simulink model "CM660A_HwTq1Meas"  (R2013b)
settings: Solver=FixedStepDiscrete  StartTime=0.0  StopTime=20  FixedStep=0.002  RelTol=1e-3
undefined symbols (not defined in the file): ELECGLBPRM_HWTQOFFS_HWNWTMTR_F32, ELECGLBPRM_HWTQSATNLOWRLIM_HWNWTMTR_F32, ELECGLBPRM_HWTQSATNUPPRLIM_HWNWTMTR_F32, ELECGLBPRM_HWTQSCA_ULS_F32, ELECGLBPRM_NOFLT_CNT_U08, ELECGLBPRM_OFFSTRIMNOTPRFM_CNT_U08, ELECGLBPRM_PRTCLFLT_CNT_U08, ELECGLBPRM_SNSRINTFLT_CNT_U08, HwTq1MeasHwTq1PrtclFltFailStep, HwTq1MeasHwTq1PrtclFltPassStep, NtcNr1, NtcSts1, RACKLIMRCCWEOTSCA_ULS_F32, RACKLIMRCWEOTSCA_ULS_F32, sigbuilder_block, SigQlfr1
libraries: simulink x25, NxtrNvM x3, NxtrLim x2
(part 1 of 3)
settings Model: RequirementInfo={'doors' '00006115' '1' 'false' 'DOORS Surrogate Item' '' } %GIDa_184d7b6b_0c7e_41d3_b9a0_1a88eb3981d4  reqMgrSettings="100 S'doors','misc'{{S'surrogatepath','savemodel','savesurrogate','updateLinks','doorsLinks2sl','slLinks2Doors','purgeDoors','purgeSimulink','detaillevel','surrogateId','synctime'{{T\"/ESG Group/CM660A_HwTq1Meas\",M[1],M[1],M[0],M[0],M[1],M[0],M[0],M[1],T\"00006115\",T\"\"}},S'mode','pathStorage'{{T\"generic\",T\"modelRelative\"}}}}"  BufferReuse=off  Creator=CZ68DS  LastModifiedBy=TZBSJD
settings SolverCC: AutoInsertRateTranBlk=on
settings DataIOCC: SaveFormat=StructureWithTime
settings OptimizationCC: BlockReduction=off  DefaultUnderspecifiedDataType=single  OptimizeBlockIOStorage=off  BufferReuse=off  ExpressionFolding=off  LocalBlockOutputs=off  OptimizeModelRefInitCode=on  LifeSpan=1
settings DebuggingCC: MultiTaskDSMMsg=warning
settings HardwareCC: ProdIntDivRoundTo=Zero  ProdEndianess=LittleEndian  ProdHWDeviceType=Generic->Custom  TargetIntDivRoundTo=Zero  TargetEndianess=LittleEndian  TargetHWDeviceType=Generic->Custom
settings RTWCC: SystemTargetFile=ert.tlc  TemplateMakefile=ert_default_tmf  Description=Embedded Coder  ProcessScript=ert_make_rtw_hook
settings CodeAppCC: IgnoreCustomStorageClasses=off
settings ERTTargetCC: CodeReplacementLibrary=ANSI_C  GenerateSampleERTMain=on  ERTCustomFileTemplate=example_file_process.tlc

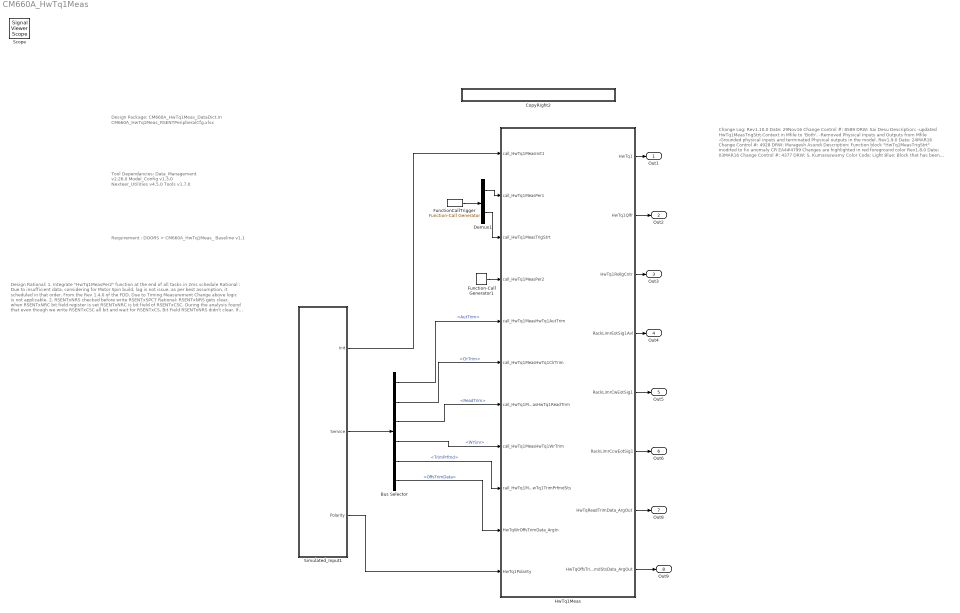
== system CM660A_HwTq1Meas ==
  note: Design Package:
      |
      | CM660A_HwTq1Meas_DataDict.m
      | CM660A_HwTq1Meas_RSENTPeripheralCfg.xlsx
  note: Change Log:
      | Rev1.10.0
      | Date: 29Nov16
      | Change Control #: 8589
      | DRW: Sai Desu
      | Description:
      | -updated HwTq1MeasTrigStrt.Context in Mfile to 'Both'.
      | -Removed Physical Inputs and Outputs from Mfile
      | -Grounded physical inputs and terminated Physical outputs in the model.
      |
      | Rev1.9.0
      | Date: 24MAR16
      | Change Control #: 4928
      | DRW: Muragesh Asundi
      | Description:
      | Function block "HwTq1MeasTrigStrt" modifed to fix anomaly CR EA4#4799
      | Changes are highlighted in red foreground color
      |
      | Rev1.8.0
      | Date: 03MAR16
      | Change Control #: 4377
      | DRW: S. Kumaraswamy
      | Color Code:
      | Light Blue:	Block that has been changed
      | 				Follow the color until the change is observed to the deepeset level
      | Dark Gray:	Client Call Blocks. Contents cannot be modified
      |
      | Rev1.7.0
      | Date: 19JAN2016
      | Change Control #: 3374
      | DRW: K. Patel
      | Description:
      | - Refer Red Color High lighted Changes.
      | - "CM660A_HwTq1Meas_RSENTPeripheralCfg.xlsx" change
      |
      | Rev1.6.0
      | Date: 16DEC2015
      | Change Control #: 3157
      | DRW: K. Patel
      | Description:
      | - Refer Red Color High lighted Changes.
      |
      | Rev: 1.5.0
      | Date: 23OCT2015
      | Change Control #: EA4#2217
      | DRW: K. Patel
      | Description:
      | - Slow Serial Message Fix
      | - EA4 Naming Correction for HwTq1MeasTrigStart
      |
      | Rev: 1.4.0
      | Date: 09OCT2015
      | Change Control #: EA4#1921
      | DRW: K. Patel
      | Description:
      | - Torque Trigger server function, Per3 change to Per2, Missing Message Counter add per1,
      | remove register from "CM660A_HwTq1Meas_RSENTPeripheralCfg.xlsx",
      | change sync time to 16
      |
      | Rev: 1.3.0
      | Date: 02OCT2015
      | Change Control #: EA4#1812
      | DRW: Pallav G/Muragesh A (KPIT)
      | Description:
      | - Corrected output signal names RickLimrCcwEotSig1,
      | RickLimrCwEotSig1 to RackLimrCcwEotSig1 and RackLimrCwEotSig1 respectively
      | - Range limiter added for above two output signals
      |
      | Rev: 1.2.0
      | Date: 20AUG2015
      | Change Control #: WCR-EA4#1285
      | DRW: K. Patel
      | Description:
      | - Rack Limiter End of Travel Signal 0 Data Read Function added
      |
      | Rev: 1.1.0
      | Date: 31JUL2015
      | Change Control #: WCR-EA4#1164
      | DRW: K. Patel
      | Description:
      | - m file correction, Tick Time change from 1us to 1.2us
      | - Global Constant
      |
      |
      | Rev: 1.0.0
      | Date: 30JUN2015
      | Change Control #: WCR-EA4#1028
      | DRW: K. Patel
      | Description:
      | - Initial Release
      | - Trim Services Added
      |
      | DRW: Keyur Patel
      | Description:
      | - Model intent to implement EA4 SENT1 based Digital Torque implementation for T1xx.
      |    model runs at three different function rate:
      |       1) Init - Configure Peripheral
      |       2) 2ms - Running SENT data, protocol fault, HwNm calculation, SENT trigger.
      |       3) 100ms - Per3 Trim Not Performed evaluation
      |       4) Event Trim Service - Auto, Clear, Write, Read, Trim Performed Status
      | - Fault Injection added
      | - Copyright Blocks added to each layer
  note: Tool Dependancies:
      |
      | Data_Management v2.26.0
      | Model_Config v1.3.0
      | Nexteer_Utilities v4.5.0
      | Tools v1.7.0
  note: Requirement :
      |
      | DOORS > CM660A_HwTq1Meas_ Baseline v1.1
  note: Design Rational:
      |
      | 1. Integrate "HwTq1MeasPer2" function at the end of all tasks in 2ms schedule
      | Rational : Due to insufficient data, considering for Motor Spin build, lag is not
      | issue, as per best assumption, it scheduled in that order.
      |
      | From the Rev 1.4.0 of the FDD, Due to Timing Measurement Change above logic
      | is not applicable.
      |
      | 2. RSENTxNRS checked before write RSENTxSPCT
      | Rational: RSENTxNRS gets clear, when RSENTxNRC bit field register is set
      | RSENTxNRC is bit field of RSENTxCSC. During the analysis found that
      | even though we write RSENTxCSC all bit and wait for RSENTxCS, Bit Field
      | RSENTxNRS didn't clear. If RSENTxNRS is set then writing RSENTxSPCT,
      | Peripheral will not output Pulse.
      |
      | Also found that RSENTxCS didn't clear itself, so need to always clear after
      | read message.
      |
      | 3. RSENTxSPCT need to write first to verify RSENTxNRS status
      | Rational : As per the Renesas User's hardware manual v1.0 -
      | Section 19 -SPC function, "Writing to RSENTnSPCT.TLL requests a
      | SPC trigger transmission. After writing to RSENTnSPCT.TLL, the CPU
      | should read RSENTnCS.NRS to check whether the previous request was
      | completed or not."
  Bus Selector : BusSelector  OutputSignals=AutTrim,ClrTrim,ReadTrim,WrSrv,TrimPrfmd,OffsTrimData
  CopyRight2 : Subsystem  Description=|  mask(Copyright Information){none=on}
      | Copyright info block.                                               
      |                                                                     
      | Place copyright information at the top of every subsystem in design.
      mask prompts: none "No parameters"
      mask help: Place copyright information at the top of every subsystem in design.
      mask Display:
      | NxtrConf = 'Nexteer Confidential';
      | 
      | sys = bdroot; %handle for the current model ("system")
      | first = get_param(sys,'Created');
      | first = first(end-3:end);  %year is last four digits
      | 
      | last = get_param(sys,'LastModifiedDate');
      | if isempty(last)
      |     last = datestr(now,'yyyy');
      | else
      |     last = last(end-3:end);
      | end
      | 
      | if strcmp(first,last)
      |     fprintf('%s -- Copyright %s Nexteer',NxtrConf,first)
      | else
      |     fprintf('%s -- %s%s- %s Nexteer',NxtrConf,char(169),first,last)
      | end
  Demux1 : Demux  Outputs=2
  Function-Call Generator1 : simulink/Ports & Subsystems/Function-Call Generator  sample_time=0.100  numberOfIterations=1
  FunctionCallTrigger : simulink/Ports & Subsystems/Function-Call Generator  RequirementInfo={} %GIDa_461051ca_e299_4da2_91c0_e73e41056377  sample_time=0.002  numberOfIterations=1
  HwTq1Meas : Subsystem  RequirementInfo={'doors' '00006115' '2' 'false' 'DOORS Surrogate Item' '' } %GIDa_76d712c1_5f1a_450e_83af_7c4f481758f4  Priority=1
      settings: AttributesFormatString=Priority = %<Priority>
  Simulated_Input1 : Subsystem  Description=Do not Code this block
      settings: AttributesFormatString=%<Description>
  Out1 : Outport
  Out2 : Outport  Port=2
  Out3 : Outport  Port=3
  Out4 : Outport  Port=4
  Out5 : Outport  Port=5
  Out6 : Outport  Port=6
  Out8 : Outport  Port=7
  Out9 : Outport  Port=8
  Scope : SignalViewerScope  IOType=viewer  RefreshTime=0.035000
  wires:
  FunctionCallTrigger/1 -> Demux1/1
  Simulated_Input1/3(Polarity) -> HwTq1Meas/11(HwTq1Polarity)
  HwTq1Meas/3(HwTq1RollgCntr) -> Out3/1
  HwTq1Meas/1(HwTq1) -> Out1/1
  HwTq1Meas/2(HwTq1Qlfr) -> Out2/1
  Function-Call Generator1/1 -> HwTq1Meas/4(call_HwTq1MeasPer2)
  Demux1/1 -> HwTq1Meas/2(call_HwTq1MeasPer1)
  Demux1/2 -> HwTq1Meas/3(call_HwTq1MeasTrigStrt)
  Bus Selector/1 -> HwTq1Meas/5(call_HwTq1MeasHwTq1AutTrim)  "<AutTrim>"
  Bus Selector/2 -> HwTq1Meas/6(call_HwTq1MeasHwTq1ClrTrim)  "<ClrTrim>"
  Bus Selector/3 -> HwTq1Meas/7(call_HwTq1MeasHwTq1ReadTrim)  "<ReadTrim>"
  Bus Selector/4 -> HwTq1Meas/8(call_HwTq1MeasHwTq1WrTrim)  "<WrSrv>"
  Bus Selector/5 -> HwTq1Meas/9(call_HwTq1MeasHwTq1TrimPrfmdSts)  "<TrimPrfmd>"
  Bus Selector/6 -> HwTq1Meas/10(HwTqWrOffsTrimData_ArgIn)  "<OffsTrimData>"
  Simulated_Input1/1(Init) -> HwTq1Meas/1(call_HwTq1MeasInit1)
  Simulated_Input1/2(Service) -> Bus Selector/1
  HwTq1Meas/4(RackLimrEotSig1Avl) -> Out4/1
  HwTq1Meas/5(RackLimrCwEotSig1) -> Out5/1
  HwTq1Meas/6(RackLimrCcwEotSig1) -> Out6/1
  HwTq1Meas/7(HwTqReadTrimData_ArgOut) -> Out8/1
  HwTq1Meas/8(HwTqOffsTrimPrfmdStsData_ArgOut) -> Out9/1

== system CM660A_HwTq1Meas/CopyRight2 ==

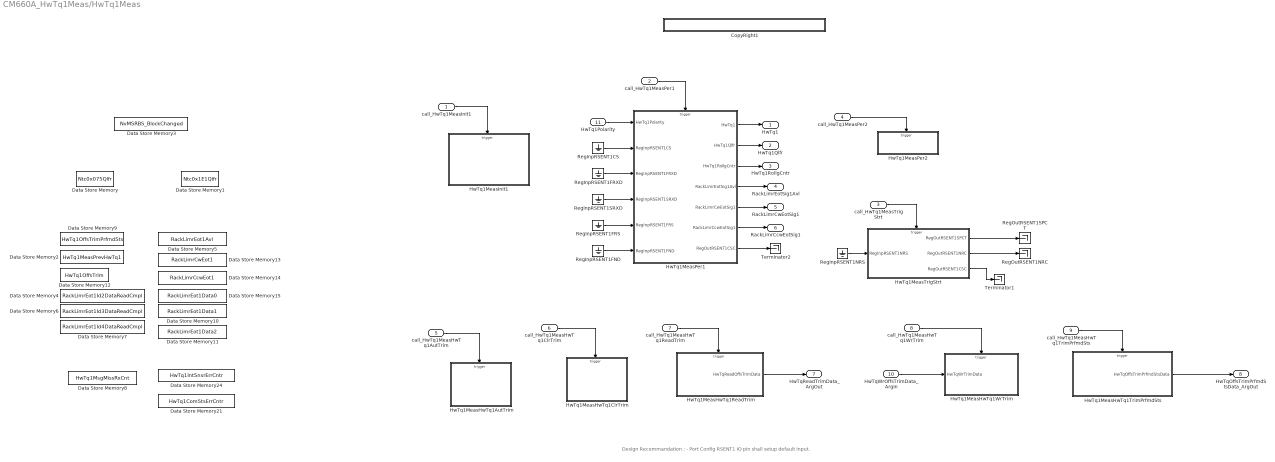
== system CM660A_HwTq1Meas/HwTq1Meas ==
  note: Design Recommandation :
      |
      | - Port Config RSENT1 IO pin shall setup default input.
  call_HwTq1MeasInit1 : Inport
  call_HwTq1MeasPer1 : Inport  Description=2ms  Port=2
      settings: AttributesFormatString=%<Description>
  call_HwTq1MeasTrigStrt : Inport  Description=Event  Port=3
      settings: AttributesFormatString=%<Description>
  call_HwTq1MeasPer2 : Inport  Description=100ms  Port=4
      settings: AttributesFormatString=%<Description>
  call_HwTq1MeasHwTq1AutTrim : Inport  Description=Event  Port=5
      settings: AttributesFormatString=%<Description>
  call_HwTq1MeasHwTq1ClrTrim : Inport  Description=Event  Port=6
      settings: AttributesFormatString=%<Description>
  call_HwTq1MeasHwTq1ReadTrim : Inport  Description=Event  Port=7
      settings: AttributesFormatString=%<Description>
  call_HwTq1MeasHwTq1WrTrim : Inport  Description=Event  Port=8
      settings: AttributesFormatString=%<Description>
  call_HwTq1MeasHwTq1TrimPrfmdSts : Inport  Description=Event  Port=9
      settings: AttributesFormatString=%<Description>
  HwTqWrOffsTrimData_ArgIn : Inport  Port=10
  HwTq1Polarity : Inport  Port=11  OutDataTypeStr=int8
  CopyRight1 : Subsystem  Description=|  mask(Copyright Information){none=on}
      | Copyright info block.                                               
      |                                                                     
      | Place copyright information at the top of every subsystem in design.
      mask prompts: none "No parameters"
      mask help: Place copyright information at the top of every subsystem in design.
      mask Display:
      | NxtrConf = 'Nexteer Confidential';
      | 
      | sys = bdroot; %handle for the current model ("system")
      | first = get_param(sys,'Created');
      | first = first(end-3:end);  %year is last four digits
      | 
      | last = get_param(sys,'LastModifiedDate');
      | if isempty(last)
      |     last = datestr(now,'yyyy');
      | else
      |     last = last(end-3:end);
      | end
      | 
      | if strcmp(first,last)
      |     fprintf('%s -- Copyright %s Nexteer',NxtrConf,first)
      | else
      |     fprintf('%s -- %s%s- %s Nexteer',NxtrConf,char(169),first,last)
      | end
  Data Store Memory10 : DataStoreMemory  DataStoreName=RackLimrEot1Data1  ReadBeforeWriteMsg=warning  WriteAfterWriteMsg=warning  WriteAfterReadMsg=warning  StateMustResolveToSignalObject=on
  Data Store Memory11 : DataStoreMemory  DataStoreName=RackLimrEot1Data2  ReadBeforeWriteMsg=warning  WriteAfterWriteMsg=warning  WriteAfterReadMsg=warning  StateMustResolveToSignalObject=on
  Data Store Memory12 : DataStoreMemory  DataStoreName=HwTq1OffsTrim  ReadBeforeWriteMsg=warning  WriteAfterWriteMsg=warning  WriteAfterReadMsg=warning
  Data Store Memory13 : DataStoreMemory  DataStoreName=RackLimrCwEot1  ReadBeforeWriteMsg=warning  WriteAfterWriteMsg=warning  WriteAfterReadMsg=warning  StateMustResolveToSignalObject=on
  Data Store Memory14 : DataStoreMemory  DataStoreName=RackLimrCcwEot1  ReadBeforeWriteMsg=warning  WriteAfterWriteMsg=warning  WriteAfterReadMsg=warning  StateMustResolveToSignalObject=on
  Data Store Memory15 : DataStoreMemory  DataStoreName=RackLimrEot1Data0  ReadBeforeWriteMsg=warning  WriteAfterWriteMsg=warning  WriteAfterReadMsg=warning  StateMustResolveToSignalObject=on
  Data Store Memory2 : DataStoreMemory  DataStoreName=HwTq1MeasPrevHwTq1  ReadBeforeWriteMsg=warning  WriteAfterWriteMsg=warning  WriteAfterReadMsg=warning
  Data Store Memory21 : DataStoreMemory  DataStoreName=HwTq1ComStsErrCntr  ReadBeforeWriteMsg=warning  WriteAfterWriteMsg=warning  WriteAfterReadMsg=warning  StateMustResolveToSignalObject=on
  Data Store Memory24 : DataStoreMemory  DataStoreName=HwTq1IntSnsrErrCntr  ReadBeforeWriteMsg=warning  WriteAfterWriteMsg=warning  WriteAfterReadMsg=warning  StateMustResolveToSignalObject=on
  Data Store Memory4 : DataStoreMemory  DataStoreName=RackLimrEot1Id2DataReadCmpl  ReadBeforeWriteMsg=warning  WriteAfterWriteMsg=warning  WriteAfterReadMsg=warning  StateMustResolveToSignalObject=on
  Data Store Memory5 : DataStoreMemory  DataStoreName=RackLimrEot1Avl  ReadBeforeWriteMsg=warning  WriteAfterWriteMsg=warning  WriteAfterReadMsg=warning  StateMustResolveToSignalObject=on
  Data Store Memory6 : DataStoreMemory  DataStoreName=RackLimrEot1Id3DataReadCmpl  ReadBeforeWriteMsg=warning  WriteAfterWriteMsg=warning  WriteAfterReadMsg=warning  StateMustResolveToSignalObject=on
  Data Store Memory7 : DataStoreMemory  DataStoreName=RackLimrEot1Id4DataReadCmpl  ReadBeforeWriteMsg=warning  WriteAfterWriteMsg=warning  WriteAfterReadMsg=warning  StateMustResolveToSignalObject=on
  Data Store Memory8 : DataStoreMemory  DataStoreName=HwTq1MsgMissRxCnt  ReadBeforeWriteMsg=warning  WriteAfterWriteMsg=warning  WriteAfterReadMsg=warning  StateMustResolveToSignalObject=on
  Data Store Memory9 : DataStoreMemory  DataStoreName=HwTq1OffsTrimPrfmdSts  ReadBeforeWriteMsg=warning  WriteAfterWriteMsg=warning  WriteAfterReadMsg=warning
  Data Store Memory : DataStoreMemory  DataStoreName=Ntc0x075Qlfr  ReadBeforeWriteMsg=warning  WriteAfterWriteMsg=warning  WriteAfterReadMsg=warning  OutDataTypeStr=uint8
      settings: AttributesFormatString=|
      | Simulation Purpose Only.
      | Do Not Code this block
      | Diagnostic Manager Owns this requirement
  Data Store Memory1 : DataStoreMemory  DataStoreName=Ntc0x1E1Qlfr  ReadBeforeWriteMsg=warning  WriteAfterWriteMsg=warning  WriteAfterReadMsg=warning  OutDataTypeStr=uint8
      settings: AttributesFormatString=|
      | Simulation Purpose Only.
      | Do Not Code this block
      | Diagnostic Manager Owns this requirement
  Data Store Memory3 : DataStoreMemory  DataStoreName=NvMSRBS_BlockChanged  ReadBeforeWriteMsg=warning  WriteAfterWriteMsg=warning  WriteAfterReadMsg=warning  OutDataTypeStr=uint8
      settings: AttributesFormatString=|
      | Simulation Purpose Only.
      | Do Not Code this block
      | Diagnostic Manager Owns this requirement
  HwTq1MeasHwTq1AutTrim : Subsystem  RequirementInfo={'doors' '00006115' '3' 'false' 'DOORS Surrogate Item' '' ; 'linktype_rmi_doors' '0000c47c (/ESG Group/FDD Module Requirements/EA4 Specific/CM660A_HwTq1Meas)' '#CM660A_56' 'true' 'REQ: CM660A_56' '' } %GIDa_78a0150d_b2b2_4893_8cf0_7a267cd87682  Priority=10  TreatAsAtomicUnit=on
      settings: AttributesFormatString=Priority=%<Priority>
  HwTq1MeasHwTq1ClrTrim : Subsystem  RequirementInfo={'doors' '00006115' '6' 'false' 'DOORS Surrogate Item' '' ; 'linktype_rmi_doors' '0000c47c (/ESG Group/FDD Module Requirements/EA4 Specific/CM660A_HwTq1Meas)' '#CM660A_54' 'true' 'REQ: CM660A_54' '' } %GIDa_9d8bf3ad_e540_4a5e_ad4c_eb940ac157ad  Priority=10  TreatAsAtomicUnit=on
      settings: AttributesFormatString=Priority=%<Priority>
  HwTq1MeasHwTq1ReadTrim : Subsystem  RequirementInfo={'doors' '00006115' '8' 'false' 'DOORS Surrogate Item' '' ; 'linktype_rmi_doors' '0000c47c (/ESG Group/FDD Module Requirements/EA4 Specific/CM660A_HwTq1Meas)' '#CM660A_52' 'true' 'REQ: CM660A_52' '' } %GIDa_4c78535b_9e38_436f_a670_46438fd62cfe  Priority=10  TreatAsAtomicUnit=on
      settings: AttributesFormatString=Priority=%<Priority>
  HwTq1MeasHwTq1TrimPrfmdSts : Subsystem  RequirementInfo={'doors' '00006115' '9' 'false' 'DOORS Surrogate Item' '' ; 'linktype_rmi_doors' '0000c47c (/ESG Group/FDD Module Requirements/EA4 Specific/CM660A_HwTq1Meas)' '#CM660A_53' 'true' 'REQ: CM660A_53' '' } %GIDa_05e70ef2_f8d5_471c_a4a3_b95d94c92180  Priority=10  TreatAsAtomicUnit=on
      settings: AttributesFormatString=Priority=%<Priority>
  HwTq1MeasHwTq1WrTrim : Subsystem  RequirementInfo={'doors' '00006115' '10' 'false' 'DOORS Surrogate Item' '' ; 'linktype_rmi_doors' '0000c47c (/ESG Group/FDD Module Requirements/EA4 Specific/CM660A_HwTq1Meas)' '#CM660A_55' 'true' 'REQ: CM660A_55' '' } %GIDa_58f23a20_9e17_4252_b727_77362ca5c7be  Priority=10  TreatAsAtomicUnit=on
      settings: AttributesFormatString=Priority=%<Priority>
  HwTq1MeasInit1 : Subsystem  TreatAsAtomicUnit=on
  HwTq1MeasPer1 : Subsystem  RequirementInfo={'doors' '00006115' '12' 'false' 'DOORS Surrogate Item' '' ; 'linktype_rmi_doors' '0000c47c (/ESG Group/FDD Module Requirements/EA4 Specific/CM660A_HwTq1Meas)' '#CM660A_27' 'true' 'REQ: CM660A_27' '' ; 'linktype_rmi_doors' '0000c47c (/ESG Group/FDD Module Requirements/EA4 Specific/CM660A_HwTq1Meas)' '#CM660A_39' 'true' 'REQ: CM660A_39' '' } %GIDa_31b3da74_5937_4fb2_b915_5c5c5e5711e7  TreatAsAtomicUnit=on
  HwTq1MeasPer2 : Subsystem  RequirementInfo={'doors' '00006115' '27' 'false' 'DOORS Surrogate Item' '' ; 'linktype_rmi_doors' '0000c47c (/ESG Group/FDD Module Requirements/EA4 Specific/CM660A_HwTq1Meas)' '#CM660A_63' 'true' 'REQ: CM660A_63' '' } %GIDa_c89b04b6_b4c1_41bf_b3f8_efad30b9fb82  Priority=8  TreatAsAtomicUnit=on
      settings: AttributesFormatString=Priority=%<Priority>
  HwTq1MeasTrigStrt : Subsystem  RequirementInfo={'doors' '00006115' '26' 'false' 'DOORS Surrogate Item' '' ; 'linktype_rmi_doors' '0000c47c (/ESG Group/FDD Module Requirements/EA4 Specific/CM660A_HwTq1Meas)' '#CM660A_33' 'true' 'REQ: CM660A_33' '' } %GIDa_ac2e4248_233e_47e7_8dc6_e55969fb5c4e  TreatAsAtomicUnit=on
  RegInpRSENT1CS : Ground
  RegInpRSENT1FND : Ground
  RegInpRSENT1FRS : Ground
  RegInpRSENT1FRXD : Ground
  RegInpRSENT1NRS : Ground
  RegInpRSENT1SRXD : Ground
  RegOutRSENT1NRC : Terminator
  RegOutRSENT1SPCT : Terminator
  Terminator1 : Terminator
  Terminator2 : Terminator
  HwTq1 : Outport
  HwTq1Qlfr : Outport  Port=2
  HwTq1RollgCntr : Outport  Port=3
  RackLimrEotSig1Avl : Outport  Port=4
  RackLimrCwEotSig1 : Outport  Port=5
  RackLimrCcwEotSig1 : Outport  Port=6
  HwTqReadTrimData_ArgOut : Outport  Port=7
  HwTqOffsTrimPrfmdStsData_ArgOut : Outport  Port=8
  wires:
  call_HwTq1MeasPer1/1 -> HwTq1MeasPer1/Trigger
  call_HwTq1MeasInit1/1 -> HwTq1MeasInit1/Trigger
  HwTq1MeasPer1/1(HwTq1) -> HwTq1/1
  HwTq1MeasPer1/2(HwTq1Qlfr) -> HwTq1Qlfr/1
  HwTq1MeasPer1/3(HwTq1RollgCntr) -> HwTq1RollgCntr/1
  call_HwTq1MeasTrigStrt/1 -> HwTq1MeasTrigStrt/Trigger
  HwTq1MeasTrigStrt/1(RegOutRSENT1SPCT) -> RegOutRSENT1SPCT/1
  call_HwTq1MeasHwTq1AutTrim/1 -> HwTq1MeasHwTq1AutTrim/Trigger
  call_HwTq1MeasHwTq1ClrTrim/1 -> HwTq1MeasHwTq1ClrTrim/Trigger
  call_HwTq1MeasHwTq1ReadTrim/1 -> HwTq1MeasHwTq1ReadTrim/Trigger
  call_HwTq1MeasHwTq1WrTrim/1 -> HwTq1MeasHwTq1WrTrim/Trigger
  call_HwTq1MeasHwTq1TrimPrfmdSts/1 -> HwTq1MeasHwTq1TrimPrfmdSts/Trigger
  HwTqWrOffsTrimData_ArgIn/1 -> HwTq1MeasHwTq1WrTrim/1(HwTqWrTrimData)
  HwTq1MeasHwTq1ReadTrim/1(HwTqReadOffsTrimData) -> HwTqReadTrimData_ArgOut/1
  HwTq1MeasHwTq1TrimPrfmdSts/1(HwTqOffsTrimPrfmdStsData) -> HwTqOffsTrimPrfmdStsData_ArgOut/1
  call_HwTq1MeasPer2/1 -> HwTq1MeasPer2/Trigger
  RegInpRSENT1CS/1 -> HwTq1MeasPer1/2(RegInpRSENT1CS)
  HwTq1MeasPer1/4(RackLimrEotSig1Avl) -> RackLimrEotSig1Avl/1
  HwTq1MeasPer1/5(RackLimrCwEotSig1) -> RackLimrCwEotSig1/1
  HwTq1MeasPer1/6(RackLimrCcwEotSig1) -> RackLimrCcwEotSig1/1
  RegInpRSENT1SRXD/1 -> HwTq1MeasPer1/4(RegInpRSENT1SRXD)
  RegInpRSENT1FRXD/1 -> HwTq1MeasPer1/3(RegInpRSENT1FRXD)
  HwTq1Polarity/1 -> HwTq1MeasPer1/1(HwTq1Polarity)
  HwTq1MeasTrigStrt/3(RegOutRSENT1CSC) -> Terminator1/1
  HwTq1MeasTrigStrt/2(RegOutRSENT1NRC) -> RegOutRSENT1NRC/1
  RegInpRSENT1NRS/1 -> HwTq1MeasTrigStrt/1(RegInpRSENT1NRS)
  HwTq1MeasPer1/7(RegOutRSENT1CSC) -> Terminator2/1
  RegInpRSENT1FRS/1 -> HwTq1MeasPer1/5(RegInpRSENT1FRS)
  RegInpRSENT1FND/1 -> HwTq1MeasPer1/6(RegInpRSENT1FND)

== system CM660A_HwTq1Meas/Simulated_Input1 ==
  Bus Creator : BusCreator  Inputs=6
  CopyRight2 : Subsystem  Description=|  mask(Copyright Information){none=on}
      | Copyright info block.                                               
      |                                                                     
      | Place copyright information at the top of every subsystem in design.
      mask prompts: none "No parameters"
      mask help: Place copyright information at the top of every subsystem in design.
      mask Display:
      | NxtrConf = 'Nexteer Confidential';
      | 
      | sys = bdroot; %handle for the current model ("system")
      | first = get_param(sys,'Created');
      | first = first(end-3:end);  %year is last four digits
      | 
      | last = get_param(sys,'LastModifiedDate');
      | if isempty(last)
      |     last = datestr(now,'yyyy');
      | else
      |     last = last(end-3:end);
      | end
      | 
      | if strcmp(first,last)
      |     fprintf('%s -- Copyright %s Nexteer',NxtrConf,first)
      | else
      |     fprintf('%s -- %s%s- %s Nexteer',NxtrConf,char(169),first,last)
      | end
  Data Type Conversion1 : DataTypeConversion  OutDataTypeStr=int8
  Data Type Conversion6 : DataTypeConversion  OutDataTypeStr=single
  Rate Transition : RateTransition
  Signal Builder : Subsystem  Tag=STV Subsys  LoadFcn=sigbuilder_block('load');  StartFcn=sigbuilder_block('start');  StopFcn=sigbuilder_block('stop');  ClipboardFcn=sigbuilder_block('clipboard');  mask(Sigbuilder block){}
      mask help: Simulink:masks:SigbuilderBlock_MD
      mask init:
      | if ~strcmp(get_param(bdroot(gcbh),'SimulationStatus'),'stopped') tuvar = sigbuilder_block('maskInit'); end
      settings: CopyFcn=sigbuilder_block('copy');  DeleteFcn=sigbuilder_block('delete');  ModelCloseFcn=sigbuilder_block('modelClose');  PreSaveFcn=sigbuilder_block('preSave');  PauseFcn=sigbuilder_block('pause');  ContinueFcn=sigbuilder_block('continue');  NameChangeFcn=sigbuilder_block('namechange');  OpenFcn=sigbuilder_block('open',[5.58621 27.931 1180.55 583.448 ]);  CloseFcn=sigbuilder_block('close');
      mask Display: plot(0, 0, 100, 100,[2, 2, 32, 32, 2], [68, 8, 8, 68, 68],[32, 2], [38, 38], [32, 19, 2],[53, 60, 44], [32, 17, 17, 2],[16, 16, 31, 31]);txt = getActiveGroup(gcbh);text(2, 100, txt,'verticalAlignment', 'top');
  Init : Outport
  Service : Outport  Port=2
  Polarity : Outport  Port=3
  wires:
  Signal Builder/8(Polarity) -> Data Type Conversion1/1  "Polarity"
  Signal Builder/1(InitTrg) -> Init/1
  Signal Builder/7(HwTqOffsTrimData) -> Data Type Conversion6/1
  Signal Builder/6(TrimPrfmdStsSrv) -> Bus Creator/5  "TrimPrfmd"
  Signal Builder/5(WrSrv) -> Bus Creator/4  "WrSrv"
  Signal Builder/4(ReadTrimSrv) -> Bus Creator/3  "ReadTrim"
  Signal Builder/3(ClearTrimSrv) -> Bus Creator/2  "ClrTrim"
  Signal Builder/2(AutTrimSrv) -> Bus Creator/1  "AutTrim"
  Bus Creator/1 -> Service/1
  Data Type Conversion1/1 -> Rate Transition/1
  Rate Transition/1 -> Polarity/1
  Data Type Conversion6/1 -> Bus Creator/6  "OffsTrimData"

== system CM660A_HwTq1Meas/HwTq1Meas/CopyRight1 ==

== system CM660A_HwTq1Meas/HwTq1Meas/HwTq1MeasHwTq1AutTrim ==
  function : TriggerPort
  CopyRight2 : Subsystem  Description=|  mask(Copyright Information){none=on}
      | Copyright info block.                                               
      |                                                                     
      | Place copyright information at the top of every subsystem in design.
      mask prompts: none "No parameters"
      mask help: Place copyright information at the top of every subsystem in design.
      mask Display:
      | NxtrConf = 'Nexteer Confidential';
      | 
      | sys = bdroot; %handle for the current model ("system")
      | first = get_param(sys,'Created');
      | first = first(end-3:end);  %year is last four digits
      | 
      | last = get_param(sys,'LastModifiedDate');
      | if isempty(last)
      |     last = datestr(now,'yyyy');
      | else
      |     last = last(end-3:end);
      | end
      | 
      | if strcmp(first,last)
      |     fprintf('%s -- Copyright %s Nexteer',NxtrConf,first)
      | else
      |     fprintf('%s -- %s%s- %s Nexteer',NxtrConf,char(169),first,last)
      | end
  NVM Shadow RAM : DataStoreWrite  RequirementInfo={} %GIDa_691c2588_2b45_48b9_9733_fd18f25444bb  DataStoreName=HwTq1OffsTrim
  NVM1 Shadow RAM : DataStoreWrite  RequirementInfo={'doors' '00006115' '4' 'false' 'DOORS Surrogate Item' '' ; 'linktype_rmi_doors' '0000c47c (/ESG Group/FDD Module Requirements/EA4 Specific/CM660A_HwTq1Meas)' '#CM660A_50' 'true' 'REQ: CM660A_50' '' } %GIDa_8dfe2b68_c9bd_4b5f_9a85_4945a725dea6  DataStoreName=HwTq1OffsTrimPrfmdSts
  PIM1 : DataStoreRead  DataStoreName=HwTq1MeasPrevHwTq1
  Set : Constant
  Set Ram Block Status : NxtrNvM/Set Ram Block Status  FuncName=Set Ram Block Status  NvMBlockName=HwTq1Offs  VoidFuncRtn=on  BlockChanged_DSN=NvMSRBS_BlockChanged  Return_DSN=NvMSRBS_Return
      settings: AttributesFormatString=%<FuncName>
  Set3 : Constant  OutDataTypeStr=uint8
  wires:
  PIM1/1 -> NVM Shadow RAM/1
  Set/1 -> NVM1 Shadow RAM/1
  Set3/1 -> Set Ram Block Status/1

== system CM660A_HwTq1Meas/HwTq1Meas/HwTq1MeasHwTq1ClrTrim ==
  function : TriggerPort
  Clear1 : Constant  Value=0  OutDataTypeStr=single
  Clear2 : Constant  Value=0
  CopyRight2 : Subsystem  Description=|  mask(Copyright Information){none=on}
      | Copyright info block.                                               
      |                                                                     
      | Place copyright information at the top of every subsystem in design.
      mask prompts: none "No parameters"
      mask help: Place copyright information at the top of every subsystem in design.
      mask Display:
      | NxtrConf = 'Nexteer Confidential';
      | 
      | sys = bdroot; %handle for the current model ("system")
      | first = get_param(sys,'Created');
      | first = first(end-3:end);  %year is last four digits
      | 
      | last = get_param(sys,'LastModifiedDate');
      | if isempty(last)
      |     last = datestr(now,'yyyy');
      | else
      |     last = last(end-3:end);
      | end
      | 
      | if strcmp(first,last)
      |     fprintf('%s -- Copyright %s Nexteer',NxtrConf,first)
      | else
      |     fprintf('%s -- %s%s- %s Nexteer',NxtrConf,char(169),first,last)
      | end
  NVM Shadow RAM : DataStoreWrite  RequirementInfo={} %GIDa_c01938bd_873a_4f20_8aad_b7368db2e426  DataStoreName=HwTq1OffsTrim
  NVM1 Shadow RAM : DataStoreWrite  RequirementInfo={'doors' '00006115' '7' 'false' 'DOORS Surrogate Item' '' ; 'linktype_rmi_doors' '0000c47c (/ESG Group/FDD Module Requirements/EA4 Specific/CM660A_HwTq1Meas)' '#CM660A_50' 'true' 'REQ: CM660A_50' '' } %GIDa_7e661117_be14_43c5_b4c7_51bd14c3b186  DataStoreName=HwTq1OffsTrimPrfmdSts
  Set Ram Block Status : NxtrNvM/Set Ram Block Status  FuncName=Set Ram Block Status  NvMBlockName=HwTq1Offs  VoidFuncRtn=on  BlockChanged_DSN=NvMSRBS_BlockChanged  Return_DSN=NvMSRBS_Return
      settings: AttributesFormatString=%<FuncName>
  Set3 : Constant  OutDataTypeStr=uint8
  wires:
  Clear1/1 -> NVM Shadow RAM/1
  Clear2/1 -> NVM1 Shadow RAM/1
  Set3/1 -> Set Ram Block Status/1

== system CM660A_HwTq1Meas/HwTq1Meas/HwTq1MeasHwTq1ReadTrim ==
  function : TriggerPort
  CopyRight2 : Subsystem  Description=|  mask(Copyright Information){none=on}
      | Copyright info block.                                               
      |                                                                     
      | Place copyright information at the top of every subsystem in design.
      mask prompts: none "No parameters"
      mask help: Place copyright information at the top of every subsystem in design.
      mask Display:
      | NxtrConf = 'Nexteer Confidential';
      | 
      | sys = bdroot; %handle for the current model ("system")
      | first = get_param(sys,'Created');
      | first = first(end-3:end);  %year is last four digits
      | 
      | last = get_param(sys,'LastModifiedDate');
      | if isempty(last)
      |     last = datestr(now,'yyyy');
      | else
      |     last = last(end-3:end);
      | end
      | 
      | if strcmp(first,last)
      |     fprintf('%s -- Copyright %s Nexteer',NxtrConf,first)
      | else
      |     fprintf('%s -- %s%s- %s Nexteer',NxtrConf,char(169),first,last)
      | end
  NVM Shadow RAM : DataStoreRead  DataStoreName=HwTq1OffsTrim
  HwTqReadOffsTrimData : Outport
  wires:
  NVM Shadow RAM/1 -> HwTqReadOffsTrimData/1

== system CM660A_HwTq1Meas/HwTq1Meas/HwTq1MeasHwTq1TrimPrfmdSts ==
  function : TriggerPort
  CopyRight2 : Subsystem  Description=|  mask(Copyright Information){none=on}
      | Copyright info block.                                               
      |                                                                     
      | Place copyright information at the top of every subsystem in design.
      mask prompts: none "No parameters"
      mask help: Place copyright information at the top of every subsystem in design.
      mask Display:
      | NxtrConf = 'Nexteer Confidential';
      | 
      | sys = bdroot; %handle for the current model ("system")
      | first = get_param(sys,'Created');
      | first = first(end-3:end);  %year is last four digits
      | 
      | last = get_param(sys,'LastModifiedDate');
      | if isempty(last)
      |     last = datestr(now,'yyyy');
      | else
      |     last = last(end-3:end);
      | end
      | 
      | if strcmp(first,last)
      |     fprintf('%s -- Copyright %s Nexteer',NxtrConf,first)
      | else
      |     fprintf('%s -- %s%s- %s Nexteer',NxtrConf,char(169),first,last)
      | end
  Data Store Read1 : DataStoreRead  DataStoreName=HwTq1OffsTrimPrfmdSts
  HwTqOffsTrimPrfmdStsData : Outport
  wires:
  Data Store Read1/1 -> HwTqOffsTrimPrfmdStsData/1

== system CM660A_HwTq1Meas/HwTq1Meas/HwTq1MeasHwTq1WrTrim ==
  HwTqWrTrimData : Inport
  function : TriggerPort
  CopyRight2 : Subsystem  Description=|  mask(Copyright Information){none=on}
      | Copyright info block.                                               
      |                                                                     
      | Place copyright information at the top of every subsystem in design.
      mask prompts: none "No parameters"
      mask help: Place copyright information at the top of every subsystem in design.
      mask Display:
      | NxtrConf = 'Nexteer Confidential';
      | 
      | sys = bdroot; %handle for the current model ("system")
      | first = get_param(sys,'Created');
      | first = first(end-3:end);  %year is last four digits
      | 
      | last = get_param(sys,'LastModifiedDate');
      | if isempty(last)
      |     last = datestr(now,'yyyy');
      | else
      |     last = last(end-3:end);
      | end
      | 
      | if strcmp(first,last)
      |     fprintf('%s -- Copyright %s Nexteer',NxtrConf,first)
      | else
      |     fprintf('%s -- %s%s- %s Nexteer',NxtrConf,char(169),first,last)
      | end
  NVM Shadow RAM : DataStoreWrite  RequirementInfo={} %GIDa_1659f01a_6b97_4ff1_afb0_e4ba99927e44  DataStoreName=HwTq1OffsTrim
  NVM1 Shadow RAM : DataStoreWrite  RequirementInfo={'doors' '00006115' '11' 'false' 'DOORS Surrogate Item' '' ; 'linktype_rmi_doors' '0000c47c (/ESG Group/FDD Module Requirements/EA4 Specific/CM660A_HwTq1Meas)' '#CM660A_50' 'true' 'REQ: CM660A_50' '' } %GIDa_340e34c7_c59a_43cb_a8d9_5aafb58ec96b  DataStoreName=HwTq1OffsTrimPrfmdSts
  Set : Constant
  Set Ram Block Status : NxtrNvM/Set Ram Block Status  FuncName=Set Ram Block Status  NvMBlockName=HwTq1Offs  VoidFuncRtn=on  BlockChanged_DSN=NvMSRBS_BlockChanged  Return_DSN=NvMSRBS_Return
      settings: AttributesFormatString=%<FuncName>
  Set3 : Constant  OutDataTypeStr=uint8
  wires:
  Set/1 -> NVM1 Shadow RAM/1
  HwTqWrTrimData/1 -> NVM Shadow RAM/1
  Set3/1 -> Set Ram Block Status/1

== system CM660A_HwTq1Meas/HwTq1Meas/HwTq1MeasInit1 ==
  note: Follow below steps in same order:
      |
      | 1. Enable Configuration mode, RSENT1MDC.OMC = 1U
      | 2. Verify whether peripheral is in Configuration mode RSENT1MST.OMS ==1U and wait till 2us* ,it is in configuration mode
      | 3. Configure the SENT Register as per  "CM660A_HwTq1Meas_RSENTPeripheralCfg.xlsx"
      | 4. Enable Operation active mode, RSENT1MDC.OMC = 5U
      | 5. Verify whether peripheral is in Opertation active mode RSENT1MST.OMS ==5U and wait till 2us* ,it is in Opertation active mode
      | 6. Client Call "IoHwAb_SetFctPrphlHwTq1"- Port Configuration shall change to output in alternate mode from default input for RSENT1 SPCO IO pin.
      |
      | Note: * - actual minimum is 150ns as per Scott Winder email from Renesas
  function : TriggerPort  TriggerType=falling
  CopyRight2 : Subsystem  Description=|  mask(Copyright Information){none=on}
      | Copyright info block.                                               
      |                                                                     
      | Place copyright information at the top of every subsystem in design.
      mask prompts: none "No parameters"
      mask help: Place copyright information at the top of every subsystem in design.
      mask Display:
      | NxtrConf = 'Nexteer Confidential';
      | 
      | sys = bdroot; %handle for the current model ("system")
      | first = get_param(sys,'Created');
      | first = first(end-3:end);  %year is last four digits
      | 
      | last = get_param(sys,'LastModifiedDate');
      | if isempty(last)
      |     last = datestr(now,'yyyy');
      | else
      |     last = last(end-3:end);
      | end
      | 
      | if strcmp(first,last)
      |     fprintf('%s -- Copyright %s Nexteer',NxtrConf,first)
      | else
      |     fprintf('%s -- %s%s- %s Nexteer',NxtrConf,char(169),first,last)
      | end
  GetRefTmr1MicroSec32bit : Subsystem
      settings: AttributesFormatString=Client Call : Start Time
  GetTiSpan1MicroSec32bit : Subsystem
  IoHwAb_SetFctPrphlHwTq1 : Subsystem
  Terminator1 : Terminator
  wires:
  GetRefTmr1MicroSec32bit/1(RefTmr) -> GetTiSpan1MicroSec32bit/1(RefTmr)
  GetTiSpan1MicroSec32bit/1(TiSpan) -> Terminator1/1

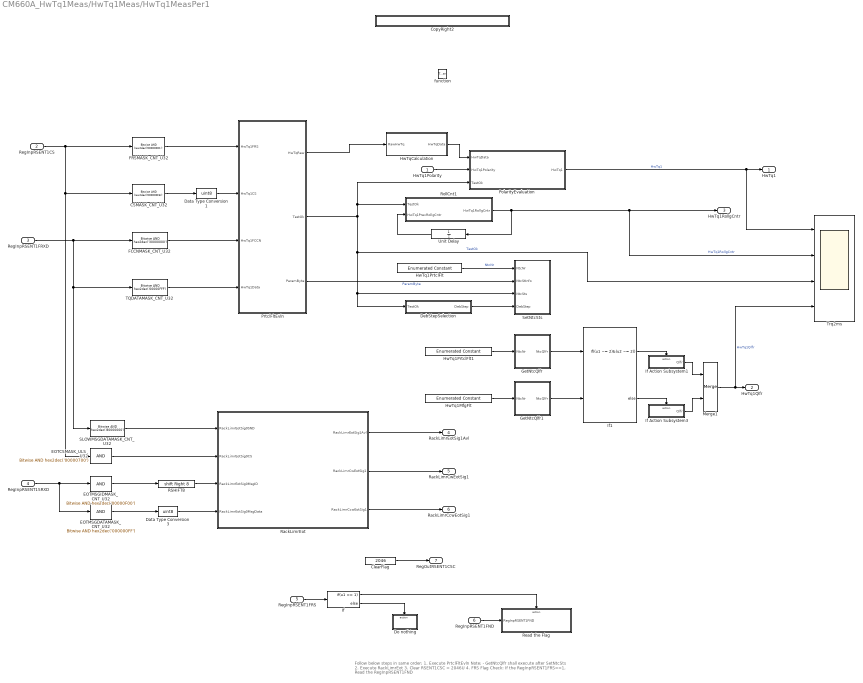
== system CM660A_HwTq1Meas/HwTq1Meas/HwTq1MeasPer1 ==
  note: Follow below steps in same order:
      |
      | 1. Execute PrtclFltEvln
      | Note: - GetNtcQlfr shall execute after SetNtcSts
      | 2. Execute RackLimrEot
      | 3. Clear RSENT1CSC = 2046U
      | 4. FRS Flag Check: If the RegInpRSENT1FRS==1,  Read the RegInpRSENT1FND
  HwTq1Polarity : Inport
  RegInpRSENT1CS : Inport  Port=2
  RegInpRSENT1FRXD : Inport  Port=3
  RegInpRSENT1SRXD : Inport  Port=4
  RegInpRSENT1FRS : Inport  Port=5
  RegInpRSENT1FND : Inport  Port=6
  function : TriggerPort  TriggerType=function-call
  CSMASK_CNT_U32 : simulink/Logic and Bit Operations/Bitwise Operator  logicop=AND  UseBitMask=on  BitMask=hex2dec('000000FE')  BitMaskRealWorld=Stored Integer
  ClearFlag : Constant  RequirementInfo={} %GIDa_f531d0e7_7b83_48fb_884c_7114bdcfdefa  Value=2046  OutDataTypeStr=uint16
  CopyRight2 : Subsystem  Description=|  mask(Copyright Information){none=on}
      | Copyright info block.                                               
      |                                                                     
      | Place copyright information at the top of every subsystem in design.
      mask prompts: none "No parameters"
      mask help: Place copyright information at the top of every subsystem in design.
      mask Display:
      | NxtrConf = 'Nexteer Confidential';
      | 
      | sys = bdroot; %handle for the current model ("system")
      | first = get_param(sys,'Created');
      | first = first(end-3:end);  %year is last four digits
      | 
      | last = get_param(sys,'LastModifiedDate');
      | if isempty(last)
      |     last = datestr(now,'yyyy');
      | else
      |     last = last(end-3:end);
      | end
      | 
      | if strcmp(first,last)
      |     fprintf('%s -- Copyright %s Nexteer',NxtrConf,first)
      | else
      |     fprintf('%s -- %s%s- %s Nexteer',NxtrConf,char(169),first,last)
      | end
  Data Type Conversion1 : DataTypeConversion  OutDataTypeStr=uint8
  Data Type Conversion3 : DataTypeConversion  OutDataTypeStr=uint8
  DebStepSelection : Subsystem
  Do nothing : Subsystem  RequirementInfo={} %GIDa_304a7da7_4af4_4490_a25d_84dbf1ee5c0e  TreatAsAtomicUnit=on
  EOTCSMASK_ULS_U32 : simulink/Logic and Bit Operations/Bitwise Operator  logicop=AND  UseBitMask=on  BitMask=hex2dec('00000700')  BitMaskRealWorld=Stored Integer
  EOTMSGDATAMASK_CNT_U32 : simulink/Logic and Bit Operations/Bitwise Operator  logicop=AND  UseBitMask=on  BitMask=hex2dec('000000FF')  BitMaskRealWorld=Stored Integer
  EOTMSGIDMASK_CNT_U32 : simulink/Logic and Bit Operations/Bitwise Operator  logicop=AND  UseBitMask=on  BitMask=hex2dec('00000F00')  BitMaskRealWorld=Stored Integer
  FCCNMASK_CNT_U32 : simulink/Logic and Bit Operations/Bitwise Operator  logicop=AND  UseBitMask=on  BitMask=hex2dec('30000000')  BitMaskRealWorld=Stored Integer
  FRSMASK_CNT_U32 : simulink/Logic and Bit Operations/Bitwise Operator  logicop=AND  UseBitMask=on  BitMask=hex2dec('00000001')  BitMaskRealWorld=Stored Integer
  GetNtcQlfr : Subsystem
  GetNtcQlfr1 : Subsystem
  HwTq1MfgFlt : simulink/Sources/Enumerated Constant  OutDataTypeStr=Enum: NtcNr1  Value=NtcNr1.NTCNR_0X1E1  SampleTime=inf
  HwTq1PrtclFlt : simulink/Sources/Enumerated Constant  OutDataTypeStr=Enum: NtcNr1  Value=NtcNr1.NTCNR_0X075  SampleTime=inf
  HwTq1PrtclFlt1 : simulink/Sources/Enumerated Constant  OutDataTypeStr=Enum: NtcNr1  Value=NtcNr1.NTCNR_0X075  SampleTime=inf
  HwTqCalculation : Subsystem
  If : If  RequirementInfo={} %GIDa_cd58525f_2a8d_4b0a_a759_5e1c1f658e4a  IfExpression=u1 == 1
  If Action Subsystem1 : Subsystem  TreatAsAtomicUnit=on
  If Action Subsystem3 : Subsystem  TreatAsAtomicUnit=on
  If1 : If  NumInputs=2  IfExpression=(u1 ~= 2)&(u2 ~= 2)
  Merge1 : Merge
  PolarityEvaluation : Subsystem  RequirementInfo={'doors' '00006115' '13' 'false' 'DOORS Surrogate Item' '' ; 'linktype_rmi_doors' '0000c47c (/ESG Group/FDD Module Requirements/EA4 Specific/CM660A_HwTq1Meas)' '#CM660A_29' 'true' 'REQ: CM660A_29' '' ; 'linktype_rmi_doors' '0000c47c (/ESG Group/FDD Module Requirements/EA4 Specific/CM660A_HwTq1Meas)' '#CM660A_32' 'true' 'REQ: CM660A_32' '' } %GIDa_7dd0f124_da9d_41af_bfd5_c8f0b8205e28
  PrtclFltEvln : Subsystem  RequirementInfo={'doors' '00006115' '16' 'false' 'DOORS Surrogate Item' '' } %GIDa_9ddede9b_2ee1_447b_ab8b_835557d5d4fb
  RSHIFT8 : ArithShift  BitShiftNumber=8  BitShiftDirection=Right
  RackLimrEot : Subsystem
  Read the Flag : Subsystem  RequirementInfo={} %GIDa_3ccebfc9_c3bd_46c1_9657_f022c7ad6929  TreatAsAtomicUnit=on
  RollCnt1 : Stateflow chart  RequirementInfo={} %GIDa_be1c412e_1791_4e7e_9b3e_cc09ba9a6629  TreatAsAtomicUnit=on
  SLOWMSGDATAMASK_CNT_U32 : simulink/Logic and Bit Operations/Bitwise Operator  logicop=AND  UseBitMask=on  BitMask=hex2dec('80000000')  BitMaskRealWorld=Stored Integer
  SetNtcSts : Subsystem  RequirementInfo={'doors' '00006115' '23' 'false' 'DOORS Surrogate Item' '' ; 'linktype_rmi_doors' '0000c47c (/ESG Group/FDD Module Requirements/EA4 Specific/CM660A_HwTq1Meas)' '#CM660A_38' 'true' 'REQ: CM660A_38' '' } %GIDa_7c28da3a_b49c_4a2c_9776_430afb4b2413
  TQDATAMASK_CNT_U32 : simulink/Logic and Bit Operations/Bitwise Operator  logicop=AND  UseBitMask=on  BitMask=hex2dec('00000FFF')  BitMaskRealWorld=Stored Integer
  Trq2ms : Scope  NumInputPorts=4
      settings: YMin=-10~0~1.9~1  YMax=10~275~2.1~2  SaveName=ScopeData3
  Unit Delay : UnitDelay  SampleTime=-1  StateName=HwTq1MeasPrevRollgCntr  StateMustResolveToSignalObject=on
      settings: AttributesFormatString=%<StateName>
  HwTq1 : Outport  RequirementInfo={} %GIDa_3b2abd0f_dff5_44f3_b788_adb2172836f5
  HwTq1Qlfr : Outport  RequirementInfo={'doors' '00006115' '24' 'false' 'DOORS Surrogate Item' '' ; 'linktype_rmi_doors' '0000c47c (/ESG Group/FDD Module Requirements/EA4 Specific/CM660A_HwTq1Meas)' '#CM660A_30' 'true' 'REQ: CM660A_30' '' } %GIDa_5eff5979_1038_44df_a727_ac7fcfb158b0  Port=2
  HwTq1RollgCntr : Outport  RequirementInfo={'doors' '00006115' '25' 'false' 'DOORS Surrogate Item' '' ; 'linktype_rmi_doors' '0000c47c (/ESG Group/FDD Module Requirements/EA4 Specific/CM660A_HwTq1Meas)' '#CM660A_31' 'true' 'REQ: CM660A_31' '' } %GIDa_de83414f_64c7_40b0_8047_6b8baba686d2  Port=3
  RackLimrEotSig1Avl : Outport  RequirementInfo={} %GIDa_12ad502d_fff8_48c8_a433_42416dc13f00  Port=4
  RackLimrCwEotSig1 : Outport  RequirementInfo={} %GIDa_86573f37_74b0_4991_9b62_ab810731bad0  Port=5
  RackLimrCcwEotSig1 : Outport  RequirementInfo={} %GIDa_8ec81f7b_3e5d_4e49_8bf0_31227f7d6107  Port=6
  RegOutRSENT1CSC : Outport  Port=7
  wires:
  PrtclFltEvln/1(HwTqRaw) -> HwTqCalculation/1(RawHwTq)
  HwTqCalculation/1(HwTqData) -> PolarityEvaluation/1(HwTqData)
  PrtclFltEvln/2(TestOk) -> PolarityEvaluation/3(TestOk), RollCnt1/1(TestOk), Trq2ms/3, SetNtcSts/3(NtcSts), DebStepSelection/1(TestOk)  "TestOk"
  HwTq1Polarity/1 -> PolarityEvaluation/2(HwTq1Polarity)
  HwTq1PrtclFlt/1 -> SetNtcSts/1(NtcNr)  "NtcNr"
  PrtclFltEvln/3(ParamByte) -> SetNtcSts/2(NtcStInfo)  "ParamByte"
  HwTq1PrtclFlt1/1 -> GetNtcQlfr/1(NtcNr)
  DebStepSelection/1(DebStep) -> SetNtcSts/4(DebStep)
  PolarityEvaluation/1(HwTq1) -> Trq2ms/1, HwTq1/1  "HwTq1"
  RollCnt1/1(HwTq1RollgCntr) -> Unit Delay/1, Trq2ms/2, HwTq1RollgCntr/1  "HwTq1RollgCntr"
  Unit Delay/1 -> RollCnt1/2(HwTq1PrevRollgCntr)
  HwTq1MfgFlt/1 -> GetNtcQlfr1/1(NtcNr)
  GetNtcQlfr/1(NtcQlfr) -> If1/1
  GetNtcQlfr1/1(NtcQlfr) -> If1/2
  If Action Subsystem1/1(Qlfr) -> Merge1/1
  If Action Subsystem3/1(Qlfr) -> Merge1/2
  Merge1/1 -> Trq2ms/4, HwTq1Qlfr/1  "HwTq1Qlfr"
  If1/2 -> If Action Subsystem3/Action
  If1/1 -> If Action Subsystem1/Action
  RackLimrEot/2(RackLimrCwEotSig1) -> RackLimrCwEotSig1/1
  RackLimrEot/3(RackLimrCcwEotSig1) -> RackLimrCcwEotSig1/1
  RackLimrEot/1(RackLimrEotSig1Avl) -> RackLimrEotSig1Avl/1
  RegInpRSENT1FRXD/1 -> TQDATAMASK_CNT_U32/1, SLOWMSGDATAMASK_CNT_U32/1, FCCNMASK_CNT_U32/1
  RegInpRSENT1CS/1 -> CSMASK_CNT_U32/1, EOTCSMASK_ULS_U32/1, FRSMASK_CNT_U32/1
  CSMASK_CNT_U32/1 -> Data Type Conversion1/1
  TQDATAMASK_CNT_U32/1 -> PrtclFltEvln/4(HwTq1Data)
  FCCNMASK_CNT_U32/1 -> PrtclFltEvln/3(HwTq1FCCN)
  FRSMASK_CNT_U32/1 -> PrtclFltEvln/1(HwTq1FRS)
  EOTCSMASK_ULS_U32/1 -> RackLimrEot/2(RackLimrEotSig0CS)
  SLOWMSGDATAMASK_CNT_U32/1 -> RackLimrEot/1(RackLimrEotSig0SND)
  RegInpRSENT1SRXD/1 -> EOTMSGDATAMASK_CNT_U32/1, EOTMSGIDMASK_CNT_U32/1
  EOTMSGIDMASK_CNT_U32/1 -> RSHIFT8/1
  EOTMSGDATAMASK_CNT_U32/1 -> Data Type Conversion3/1
  RSHIFT8/1 -> RackLimrEot/3(RackLimrEotSig0MsgID)
  Data Type Conversion3/1 -> RackLimrEot/4(RackLimrEotSig0MsgData)
  Data Type Conversion1/1 -> PrtclFltEvln/2(HwTq1CS)
  RegInpRSENT1FRS/1 -> If/1
  If/1 -> Read the Flag/Action
  If/2 -> Do nothing/Action
  RegInpRSENT1FND/1 -> Read the Flag/1(RegInpRSENT1FND)
  ClearFlag/1 -> RegOutRSENT1CSC/1

== system CM660A_HwTq1Meas/HwTq1Meas/HwTq1MeasPer2 ==
  note: Information Only:
      | - Trim not performed Ntc
  function : TriggerPort  TriggerType=function-call
  CopyRight2 : Subsystem  Description=|  mask(Copyright Information){none=on}
      | Copyright info block.                                               
      |                                                                     
      | Place copyright information at the top of every subsystem in design.
      mask prompts: none "No parameters"
      mask help: Place copyright information at the top of every subsystem in design.
      mask Display:
      | NxtrConf = 'Nexteer Confidential';
      | 
      | sys = bdroot; %handle for the current model ("system")
      | first = get_param(sys,'Created');
      | first = first(end-3:end);  %year is last four digits
      | 
      | last = get_param(sys,'LastModifiedDate');
      | if isempty(last)
      |     last = datestr(now,'yyyy');
      | else
      |     last = last(end-3:end);
      | end
      | 
      | if strcmp(first,last)
      |     fprintf('%s -- Copyright %s Nexteer',NxtrConf,first)
      | else
      |     fprintf('%s -- %s%s- %s Nexteer',NxtrConf,char(169),first,last)
      | end
  Data Store Read1 : DataStoreRead  DataStoreName=HwTq1OffsTrimPrfmdSts
  Ground : Ground
  If : If  IfExpression=(u1 ~= 0)
  If Action Subsystem : Subsystem  RequirementInfo={'doors' '00006115' '28' 'false' 'DOORS Surrogate Item' '' ; 'linktype_rmi_doors' '0000c47c (/ESG Group/FDD Module Requirements/EA4 Specific/CM660A_HwTq1Meas)' '#CM660A_67' 'true' 'REQ: CM660A_67' '' } %GIDa_eda0e9fe_0ef4_4d37_918c_815346a1604f  TreatAsAtomicUnit=on
  If Action Subsystem1 : Subsystem  RequirementInfo={'doors' '00006115' '29' 'false' 'DOORS Surrogate Item' '' ; 'linktype_rmi_doors' '0000c47c (/ESG Group/FDD Module Requirements/EA4 Specific/CM660A_HwTq1Meas)' '#CM660A_65' 'true' 'REQ: CM660A_65' '' } %GIDa_f1a05e9a_fff8_4eab_8b85_2e72f495a740  TreatAsAtomicUnit=on
  Merge : Merge
  Merge1 : Merge
  NtcNr : simulink/Sources/Enumerated Constant  OutDataTypeStr=Enum: NtcNr1  Value=NtcNr1.NTCNR_0X1E1  SampleTime=inf
  Scope : Scope  NumInputPorts=2
      settings: YMin=-5~-5  YMax=5~5  SaveName=ScopeData3
  SetNtcSts : Subsystem  RequirementInfo={'doors' '00006115' '30' 'false' 'DOORS Surrogate Item' '' ; 'linktype_rmi_doors' '0000c47c (/ESG Group/FDD Module Requirements/EA4 Specific/CM660A_HwTq1Meas)' '#CM660A_61' 'true' 'REQ: CM660A_61' '' } %GIDa_03dde2fd_062f_4b23_859a_fc5579118954
  wires:
  Ground/1 -> SetNtcSts/4(DebStep)
  NtcNr/1 -> SetNtcSts/1(NtcNr)
  Data Store Read1/1 -> If/1
  If/1 -> If Action Subsystem/Action
  If/2 -> If Action Subsystem1/Action
  If Action Subsystem/1(ParamByte) -> Merge/1
  If Action Subsystem1/1(ParamByte) -> Merge/2
  If Action Subsystem/2(TestOk) -> Merge1/1
  If Action Subsystem1/2(TestOk) -> Merge1/2
  Merge/1 -> Scope/1, SetNtcSts/2(NtcStInfo)  "ParamByte"
  Merge1/1 -> Scope/2, SetNtcSts/3(NtcSts)  "TestOk"

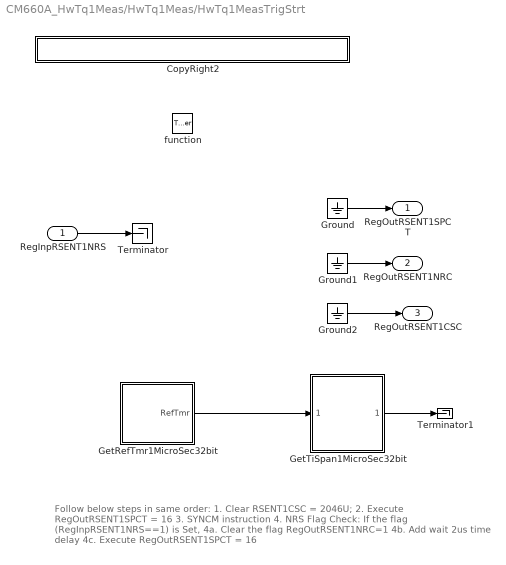
== system CM660A_HwTq1Meas/HwTq1Meas/HwTq1MeasTrigStrt ==
  note: Follow below steps in same order:
      |
      | 1. Clear RSENT1CSC = 2046U;
      | 2. Execute RegOutRSENT1SPCT = 16
      | 3. SYNCM instruction
      |
      | 4. NRS Flag Check: If the flag (RegInpRSENT1NRS==1) is Set,
      | 	4a. Clear the flag RegOutRSENT1NRC=1
      | 	4b. Add wait 2us time delay
      | 	4c. Execute RegOutRSENT1SPCT = 16
  RegInpRSENT1NRS : Inport
  function : TriggerPort  TriggerType=function-call
  CopyRight2 : Subsystem  Description=|  mask(Copyright Information){none=on}
      | Copyright info block.                                               
      |                                                                     
      | Place copyright information at the top of every subsystem in design.
      mask prompts: none "No parameters"
      mask help: Place copyright information at the top of every subsystem in design.
      mask Display:
      | NxtrConf = 'Nexteer Confidential';
      | 
      | sys = bdroot; %handle for the current model ("system")
      | first = get_param(sys,'Created');
      | first = first(end-3:end);  %year is last four digits
      | 
      | last = get_param(sys,'LastModifiedDate');
      | if isempty(last)
      |     last = datestr(now,'yyyy');
      | else
      |     last = last(end-3:end);
      | end
      | 
      | if strcmp(first,last)
      |     fprintf('%s -- Copyright %s Nexteer',NxtrConf,first)
      | else
      |     fprintf('%s -- %s%s- %s Nexteer',NxtrConf,char(169),first,last)
      | end
  GetRefTmr1MicroSec32bit : Subsystem
      settings: AttributesFormatString=Client Call : Start Time
  GetTiSpan1MicroSec32bit : Subsystem
  Ground : Ground
  Ground1 : Ground
  Ground2 : Ground
  Terminator : Terminator
  Terminator1 : Terminator
  RegOutRSENT1SPCT : Outport
  RegOutRSENT1NRC : Outport  Port=2
  RegOutRSENT1CSC : Outport  Port=3
  wires:
  ? -> ?
  Ground1/1 -> RegOutRSENT1NRC/1
  Ground/1 -> RegOutRSENT1SPCT/1
  Ground2/1 -> RegOutRSENT1CSC/1
  RegInpRSENT1NRS/1 -> Terminator/1
  GetTiSpan1MicroSec32bit/1(TiSpan) -> Terminator1/1
  GetRefTmr1MicroSec32bit/1(RefTmr) -> GetTiSpan1MicroSec32bit/1(RefTmr)

== system CM660A_HwTq1Meas/Simulated_Input1/CopyRight2 ==

== system CM660A_HwTq1Meas/Simulated_Input1/Signal Builder ==
  Demux : Demux  Tag=STV Demux  Outputs=8
  FromWs : FromWorkspace  Tag=STV FromWs  VariableName=tuvar  SampleTime=0  OutputAfterFinalValue=Holding final value
      SigBuilderData=|
      | common.afterFinalStr = 'Hold final value'
      | common.sampleTime = '0'
      | dataSet(1).timeRange = [0 20]
      | dataSet(1).name = 'IdealSignal'
      | dataSet(2).timeRange = [0 20]
      | dataSet(2).name = 'Faults'
      | dataSet(3).timeRange = [0 20]
      | dataSet(3).name = 'Service'
      | sbobj.Groups(1).Name = 'IdealSignal'
      | sbobj.Groups(1).Signals(1).Name = 'InitTrg'
      | sbobj.Groups(1).Signals(1).XData = [0 0.02 0.02 0.06 0.06 20]
      | sbobj.Groups(1).Signals(1).YData = [0 0 1 1 0 0]
      | sbobj.Groups(1).Signals(2).Name = 'AutTrimSrv'
      | sbobj.Groups(1).Signals(2).XData = [0 20]
      | sbobj.Groups(1).Signals(2).YData = [0 0]
      | sbobj.Groups(1).Signals(3).Name = 'ClearTrimSrv'
      | sbobj.Groups(1).Signals(3).XData = [0 20]
      | sbobj.Groups(1).Signals(3).YData = [0 0]
      | sbobj.Groups(1).Signals(4).Name = 'ReadTrimSrv'
      | sbobj.Groups(1).Signals(4).XData = [0 20]
      | sbobj.Groups(1).Signals(4).YData = [0 0]
      | sbobj.Groups(1).Signals(5).Name = 'WrSrv'
      | sbobj.Groups(1).Signals(5).XData = [0 0.04 0.04 0.08 0.08 20]
      | sbobj.Groups(1).Signals(5).YData = [0 0 1 1 0 0]
      | sbobj.Groups(1).Signals(6).Name = 'TrimPrfmdStsSrv'
      | sbobj.Groups(1).Signals(6).XData = [0 20]
      | sbobj.Groups(1).Signals(6).YData = [0 0]
      | sbobj.Groups(1).Signals(7).Name = 'HwTqOffsTrimData'
      | sbobj.Groups(1).Signals(7).XData = [0 20]
      | sbobj.Groups(1).Signals(7).YData = [0 0]
      | sbobj.Groups(1).Signals(8).Name = 'Polarity'
      | sbobj.Groups(1).Signals(8).XData = [0 20]
      | sbobj.Groups(1).Signals(8).YData = [1 1]
      | sbobj.Groups(1).TimeRange = [0 20]
      | sbobj.Groups(2).Name = 'Faults'
      | sbobj.Groups(2).Signals(1).Name = 'InitTrg'
      | sbobj.Groups(2).Signals(1).XData = [0 0.02 0.02 0.06 0.06 20]
      | sbobj.Groups(2).Signals(1).YData = [0 0 1 1 0 0]
      | sbobj.Groups(2).Signals(2).Name = 'AutTrimSrv'
      | sbobj.Groups(2).Signals(2).XData = [0 20]
      | sbobj.Groups(2).Signals(2).YData = [0 0]
      | sbobj.Groups(2).Signals(3).Name = 'ClearTrimSrv'
      | sbobj.Groups(2).Signals(3).XData = [0 20]
      | sbobj.Groups(2).Signals(3).YData = [0 0]
      | sbobj.Groups(2).Signals(4).Name = 'ReadTrimSrv'
      | sbobj.Groups(2).Signals(4).XData = [0 20]
      | sbobj.Groups(2).Signals(4).YData = [0 0]
      | sbobj.Groups(2).Signals(5).Name = 'WrSrv'
      | sbobj.Groups(2).Signals(5).XData = [0 0.06 0.06 0.12 0.12 20]
      | sbobj.Groups(2).Signals(5).YData = [0 0 1 1 0 0]
      | sbobj.Groups(2).Signals(6).Name = 'TrimPrfmdStsSrv'
      | sbobj.Groups(2).Signals(6).XData = [0 20]
      | sbobj.Groups(2).Signals(6).YData = [0 0]
      | sbobj.Groups(2).Signals(7).Name = 'HwTqOffsTrimData'
      | sbobj.Groups(2).Signals(7).XData = [0 20]
      | sbobj.Groups(2).Signals(7).YData = [0 0]
      | sbobj.Groups(2).Signals(8).Name = 'Polarity'
      | sbobj.Groups(2).Signals(8).XData = [0 11 11 20]
      | sbobj.Groups(2).Signals(8).YData = [-1 -1 1 1]
      | sbobj.Groups(2).TimeRange = [0 20]
      | sbobj.Groups(3).Name = 'Service'
      | sbobj.Groups(3).Signals(1).Name = 'InitTrg'
      | sbobj.Groups(3).Signals(1).XData = [0 0.02 0.02 0.06 0.06 20]
      | sbobj.Groups(3).Signals(1).YData = [0 0 1 1 0 0]
      | sbobj.Groups(3).Signals(2).Name = 'AutTrimSrv'
      | sbobj.Groups(3).Signals(2).XData = [0 0.58 0.58 0.68 0.68 16 16 16.1 16.1 20]
      | sbobj.Groups(3).Signals(2).YData = [0 0 1 1 0 0 1 1 0 0]
      | sbobj.Groups(3).Signals(3).Name = 'ClearTrimSrv'
      | sbobj.Groups(3).Signals(3).XData = [0 0.34 4.1 4.1 4.16 4.16 9.98 9.98 10.06 10.06 20]
      | sbobj.Groups(3).Signals(3).YData = [0 0 0 1 1 0 0 1 1 0 0]
      | sbobj.Groups(3).Signals(4).Name = 'ReadTrimSrv'
      | sbobj.Groups(3).Signals(4).XData = [0 1.24 1.24 1.32 1.32 4.62 4.62 4.7 4.7 6.84 6.84 6.92 6.92 10.38 10.38 10.46 10.46 16.72 16.72 16.8 16.8 20]
      | sbobj.Groups(3).Signals(4).YData = [0 0 1 1 0 0 1 1 0 0 1 1 0 0 1 1 0 0 1 1 0 0]
      | sbobj.Groups(3).Signals(5).Name = 'WrSrv'
      | sbobj.Groups(3).Signals(5).XData = [0 6.22 6.22 6.3 6.3 20]
      | sbobj.Groups(3).Signals(5).YData = [0 0 1 1 0 0]
      | sbobj.Groups(3).Signals(6).Name = 'TrimPrfmdStsSrv'
      | sbobj.Groups(3).Signals(6).XData = [0 1.24 1.24 1.32 1.32 4.64 4.64 4.7 4.7 6.84 6.84 6.92 6.92 10.64 10.64 10.72 10.72 16.74 16.74 16.82 16.82 20]
      | sbobj.Groups(3).Signals(6).YData = [0 0 1 1 0 0 1 1 0 0 1 1 0 0 1 1 0 0 1 1 0 0]
      | sbobj.Groups(3).Signals(7).Name = 'HwTqOffsTrimData'
      | sbobj.Groups(3).Signals(7).XData = [0 0.4 5.78 5.78 7.62 7.62 20]
      | sbobj.Groups(3).Signals(7).YData = [0 0 0 5 5 0 0]
      | sbobj.Groups(3).Signals(8).Name = 'Polarity'
      | sbobj.Groups(3).Signals(8).XData = [0 20]
      | sbobj.Groups(3).Signals(8).YData = [1 1]
      | sbobj.Groups(3).TimeRange = [0 20]
  InitTrg : Outport  Tag=STV Outport
  AutTrimSrv : Outport  Tag=STV Outport  Port=2
  ClearTrimSrv : Outport  Tag=STV Outport  Port=3
  ReadTrimSrv : Outport  Tag=STV Outport  Port=4
  WrSrv : Outport  Tag=STV Outport  Port=5
  TrimPrfmdStsSrv : Outport  Tag=STV Outport  Port=6
  HwTqOffsTrimData : Outport  Tag=STV Outport  Port=7
  Polarity : Outport  Tag=STV Outport  Port=8
  wires:
  Demux/8 -> Polarity/1
  Demux/7 -> HwTqOffsTrimData/1
  Demux/6 -> TrimPrfmdStsSrv/1
  Demux/5 -> WrSrv/1
  Demux/4 -> ReadTrimSrv/1
  Demux/3 -> ClearTrimSrv/1
  Demux/2 -> AutTrimSrv/1
  Demux/1 -> InitTrg/1
  FromWs/1 -> Demux/1

== system CM660A_HwTq1Meas/HwTq1Meas/HwTq1MeasHwTq1AutTrim/CopyRight2 ==

== system CM660A_HwTq1Meas/HwTq1Meas/HwTq1MeasHwTq1ClrTrim/CopyRight2 ==

== system CM660A_HwTq1Meas/HwTq1Meas/HwTq1MeasHwTq1ReadTrim/CopyRight2 ==

== system CM660A_HwTq1Meas/HwTq1Meas/HwTq1MeasHwTq1TrimPrfmdSts/CopyRight2 ==

== system CM660A_HwTq1Meas/HwTq1Meas/HwTq1MeasHwTq1WrTrim/CopyRight2 ==

== system CM660A_HwTq1Meas/HwTq1Meas/HwTq1MeasInit1/CopyRight2 ==
